simulink model "sim_translation_guidance_law"  (R2024b)
settings: Solver=ode4  StartTime=0.0  StopTime=5000  FixedStep=0.01  RelTol=1e-3
values from neighbouring files (symbols this model uses):
  at_approach = [ax2_t; ay2_t; az2_t]    [guidance_law.m]
  g_moon = 1.62    [guidance_law.m]
  masses = masses(:)    [total_inertia.m]
  r0 = [x0; y0; z0]    [guidance_law.m]
  rt_approach = [x2_t; y2_t; z2_t]    [guidance_law.m]
  rt_breaking = [x1_t; y1_t; z1_t]    [guidance_law.m]
  tgo_approach = 150    [guidance_law.m]
  tgo_breaking = Tgo1    [guidance_law.m]
  v0 = [vx0; vy0; vz0]    [guidance_law.m]
  vt_approach = [vx2_t; vy2_t; vz2_t]    [guidance_law.m]
  vt_breaking = [vx1_t; vy1_t; vz1_t]    [guidance_law.m]
undefined symbols (not defined in the file or in its folder): LLM
libraries: simulink x1
settings Model: NumberOfSteps=2  Creator=gabri  LastModifiedBy=gabri

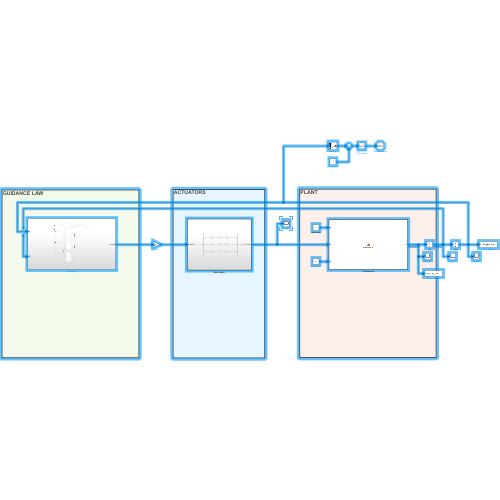
[thumbnail: Simulink's stored preview of the top-level diagram]
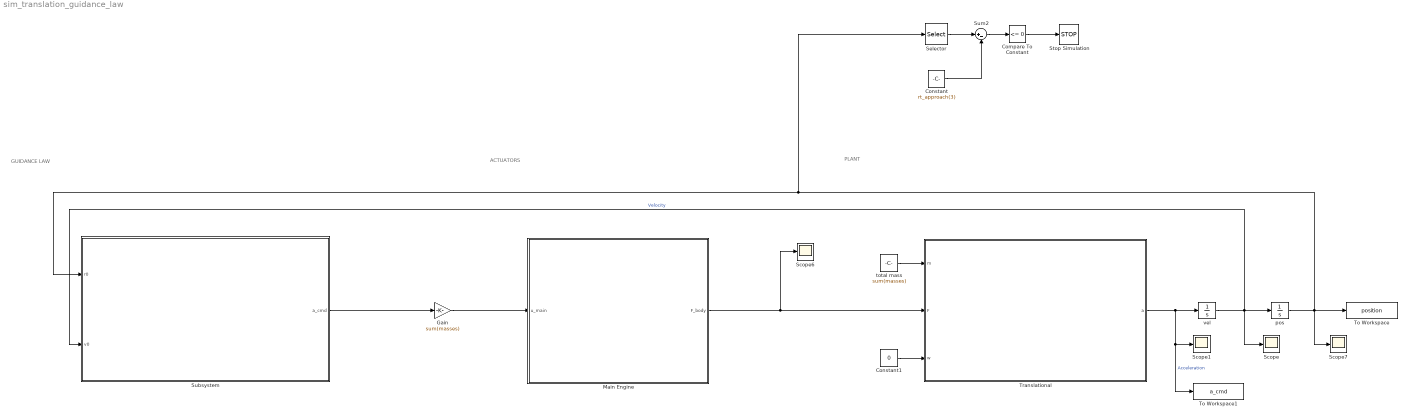
== system sim_translation_guidance_law ==
  note: ACTUATORS
  note: PLANT
  note: GUIDANCE LAW
  Compare To Constant : simulink/Logic and Bit Operations/Compare To Constant  relop=<=  const=0  OutDataTypeStr=boolean
  Constant : Constant  Value=rt_approach(3)
  Constant1 : Constant  Value=0
  Gain : Gain  Gain=sum(masses)
  Main Engine : Subsystem  TreatAsAtomicUnit=on
  Scope{,1,6..7} (4 alike) : Scope
  Selector : Selector  InputPortWidth=3  IndexOptions=Index vector (dialog)  Indices=[3]  OutputSizes=1
  Stop Simulation : Stop
  Subsystem : Subsystem
  Sum2 : Sum  Inputs=|+-
  To Workspace : ToWorkspace  VariableName=position  SampleTime=-1
  To Workspace1 : ToWorkspace  VariableName=a_cmd  SampleTime=-1
  Translational : MATLAB Function  TreatAsAtomicUnit=on
  pos : Integrator  InitialCondition=r0
  total mass : Constant  Value=sum(masses)
  vel : Integrator  InitialCondition=v0
  wires:
  vel/1 -> Subsystem/2(v0), pos/1, Scope/1  "Velocity"
  Main Engine/1(F_body) -> Scope6/1, Translational/2(F)
  Constant1/1 -> Translational/3(w)
  total mass/1 -> Translational/1(m)
  Translational/1(a) -> vel/1, To Workspace1/1, Scope1/1  "Acceleration"
  pos/1 -> Subsystem/1(r0), Selector/1, To Workspace/1, Scope7/1
  Subsystem/1(a_cmd) -> Gain/1
  Gain/1 -> Main Engine/1(u_main)
  Compare To Constant/1 -> Stop Simulation/1
  Sum2/1 -> Compare To Constant/1
  Constant/1 -> Sum2/2
  Selector/1 -> Sum2/1

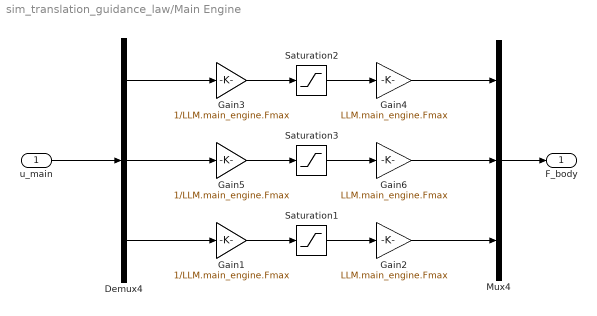
== system sim_translation_guidance_law/Main Engine ==
  u_main : Inport
  Demux4 : Demux  Outputs=3
  Gain1 : Gain  Gain=1/LLM.main_engine.Fmax
  Gain2 : Gain  Gain=LLM.main_engine.Fmax
  Gain3 : Gain  Gain=1/LLM.main_engine.Fmax
  Gain4 : Gain  Gain=LLM.main_engine.Fmax
  Gain5 : Gain  Gain=1/LLM.main_engine.Fmax
  Gain6 : Gain  Gain=LLM.main_engine.Fmax
  Mux4 : Mux  Inputs=3
  Saturation1 : Saturate  UpperLimit=1  LowerLimit=-1
  Saturation2 : Saturate  UpperLimit=1  LowerLimit=-1
  Saturation3 : Saturate  UpperLimit=1  LowerLimit=-1
  F_body : Outport
  wires:
  Demux4/3 -> Gain1/1
  u_main/1 -> Demux4/1
  Mux4/1 -> F_body/1
  Gain2/1 -> Mux4/3
  Saturation1/1 -> Gain2/1
  Gain1/1 -> Saturation1/1
  Gain4/1 -> Mux4/1
  Demux4/1 -> Gain3/1
  Saturation2/1 -> Gain4/1
  Gain3/1 -> Saturation2/1
  Gain6/1 -> Mux4/2
  Demux4/2 -> Gain5/1
  Saturation3/1 -> Gain6/1
  Gain5/1 -> Saturation3/1

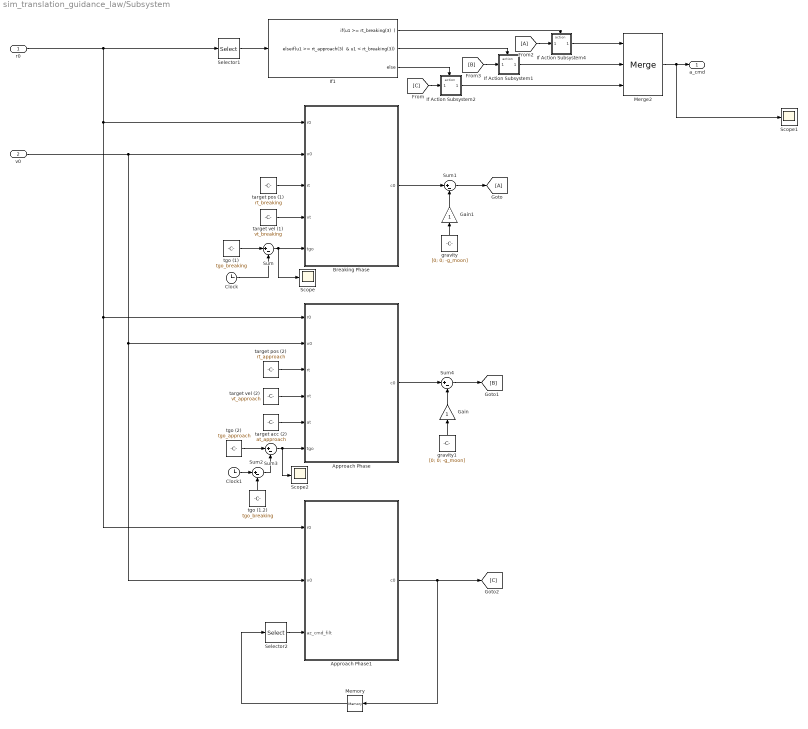
== system sim_translation_guidance_law/Subsystem ==
  r0 : Inport
  v0 : Inport  Port=2
  Approach Phase : MATLAB Function  TreatAsAtomicUnit=on
  Approach Phase1 : MATLAB Function  TreatAsAtomicUnit=on
  Breaking Phase : MATLAB Function  TreatAsAtomicUnit=on
  Clock : Clock
  Clock1 : Clock
  From2 : From
  Gain : Gain
  Gain1 : Gain
  Goto : Goto
  If Action Subsystem1 : Subsystem  TreatAsAtomicUnit=on
  If Action Subsystem2 : Subsystem  TreatAsAtomicUnit=on
  If Action Subsystem4 : Subsystem  TreatAsAtomicUnit=on
  If1 : If  IfExpression=u1 >= rt_breaking(3)  ElseIfExpressions="u1 >= rt_approach(3)  & u1 < rt_breaking(3)"
  Memory : Memory
  Merge2 : Merge  Inputs=3
  Scope : Scope
  Scope1 : Scope
  Scope2 : Scope
  Selector1 : Selector  InputPortWidth=3  IndexOptions=Index vector (dialog)  Indices=[3]  OutputSizes=1
  Selector2 : Selector  InputPortWidth=3  IndexOptions=Index vector (dialog)  Indices=[3]  OutputSizes=1
  Sum{,1..4} (5 alike) : Sum  Inputs=|+-
  gravity : Constant  Value=[0; 0; -g_moon]
  gravity1 : Constant  Value=[0; 0; -g_moon]
  target acc (2) : Constant  Value=at_approach
  target pos (1) : Constant  Value=rt_breaking
  target pos (2) : Constant  Value=rt_approach
  target vel (1) : Constant  Value=vt_breaking
  target vel (2) : Constant  Value=vt_approach
  tgo (1) : Constant  Value=tgo_breaking
  tgo (1.2) : Constant  Value=tgo_breaking
  tgo (2) : Constant  Value=tgo_approach
  a_cmd : Outport
  wires:
  r0/1 -> Approach Phase1/1(r0), Approach Phase/1(r0), Breaking Phase/1(r0), Selector1/1
  v0/1 -> Approach Phase1/2(v0), Approach Phase/2(v0), Breaking Phase/2(v0)
  target vel (1)/1 -> Breaking Phase/4(vt)
  target pos (1)/1 -> Breaking Phase/3(rt)
  Clock/1 -> Sum/2
  tgo (1)/1 -> Sum/1
  Sum/1 -> Scope/1, Breaking Phase/5(tgo)
  Breaking Phase/1(c0) -> Sum1/1
  gravity/1 -> Gain1/1
  Sum1/1 -> Goto/1
  Sum3/1 -> Approach Phase/6(tgo), Scope2/1
  tgo (2)/1 -> Sum3/1
  Selector1/1 -> If1/1
  target pos (2)/1 -> Approach Phase/3(rt)
  target vel (2)/1 -> Approach Phase/4(vt)
  target acc (2)/1 -> Approach Phase/5(at)
  Sum4/1 -> [B]
  Approach Phase/1(c0) -> Sum4/1
  gravity1/1 -> Gain/1
  [B] -> If Action Subsystem1/1(a_cmd)
  From2/1 -> If Action Subsystem4/1(a_cmd)
  If Action Subsystem1/1(Out1) -> Merge2/2
  If Action Subsystem4/1(Out1) -> Merge2/1
  Merge2/1 -> Scope1/1, a_cmd/1
  If1/1 -> If Action Subsystem4/Action
  Clock1/1 -> Sum2/1
  Sum2/1 -> Sum3/2
  tgo (1.2)/1 -> Sum2/2
  If1/2 -> If Action Subsystem1/Action
  If1/3 -> If Action Subsystem2/Action
  If Action Subsystem2/1(a_cmd) -> Merge2/3
  Approach Phase1/1(c0) -> Memory/1, [C]
  [C] -> If Action Subsystem2/1(Input)
  Selector2/1 -> Approach Phase1/3(az_cmd_filt)
  Memory/1 -> Selector2/1
  Gain/1 -> Sum4/2
  Gain1/1 -> Sum1/2

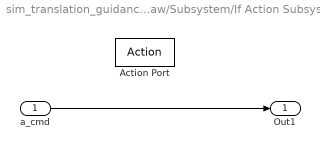
== system sim_translation_guidance_law/Subsystem/If Action Subsystem1 ==
  a_cmd : Inport
  Action Port : ActionPort  ActionPortLabel="elseif(u1 >= rt_approach(3)  & u1 < rt_breaking(3)  )"
  Out1 : Outport
  wires:
  a_cmd/1 -> Out1/1

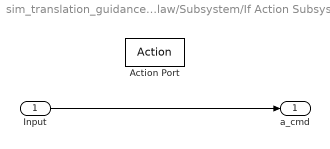
== system sim_translation_guidance_law/Subsystem/If Action Subsystem2 ==
  Input : Inport
  Action Port : ActionPort  ActionPortLabel=else
  a_cmd : Outport
  wires:
  Input/1 -> a_cmd/1

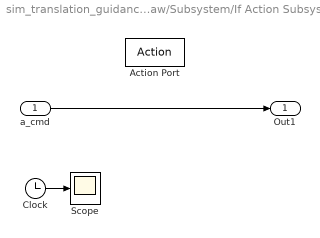
== system sim_translation_guidance_law/Subsystem/If Action Subsystem4 ==
  a_cmd : Inport
  Action Port : ActionPort  ActionPortLabel="if(u1 >= rt_breaking(3)  )"
  Clock : Clock
  Scope : Scope
  Out1 : Outport
  wires:
  a_cmd/1 -> Out1/1
  Clock/1 -> Scope/1

== matlab function sim_translation_guidance_law/Subsystem/Approach Phase ==
  data: r0 input; c0 output; v0 input; rt input; vt input; at input; tgo input
function c0 = approach_coeffs(r0,v0,rt,vt,at,tgo)

    c0 = at - 6*(vt+v0)/tgo + 12*(rt - r0)/(tgo^2);
    if tgo<1
        tgo = 1;
        c0 = [0; 0; -1.63];
    end

end

== matlab function sim_translation_guidance_law/Subsystem/Breaking Phase ==
  data: r0 input; c0 output; v0 input; rt input; vt input; tgo input
function c0 = braking_coeffs(r0, v0, rt, vt, tgo)
    
    c0 = (-2*(vt+2*v0))/tgo + 6*(rt - r0)/(tgo^2);
    if tgo<0.5
        c0 = [0; 0; -1.63];
    end

end

== matlab function sim_translation_guidance_law/Subsystem/Approach Phase1 ==
  data: r0 input; c0 output; v0 input; az_cmd_filt input
function c0 = approach_coeffs(r0,v0,az_cmd_filt)
    
    g_moon  = 1.62;
    az3_cmd = 1.2*g_moon;

    clip = @(u,umin,umax) max(min(u,umax),umin);

    if ~exist('Kxy','var'),      Kxy = 0.8; end
    if ~exist('ax_max','var'),   ax_max = 2.0; end
    if ~exist('ay_max','var'),   ay_max = 2.0; end
    if ~exist('daz_max','var'),  daz_max = 0.6*g_moon; end
    if ~exist('az_cmd_filt','var'), az_cmd_filt = az3_cmd; end
    
    v_td   = -0.1;                 % m/s target at impact
    az_nom = az3_cmd;              % m/s^2 (1.2 g_moon)
    az_max = az_nom + daz_max;     % thrust bound
    a_up_max = max(az_max - g_moon, 0.1);  % net braking capability
    alpha_f  = 0.6;                % smoothing 0..1
    
    % (2) DIVERT table (from your table)
    divert_D   = [25   50    75   100   125   150];      % m
    divert_dT  = [-0.9 -0.6  4.0   8.3   11.1  15.4];    % s
    divert_dDV = [-0.9  0.6  8.2  15.5   20.3  27.4];    % m/s (info)
    
    % Additional remaining time (decreases over time)
    dT_hold = 0;    % s
    dDV_est = 0;    % m/s (optional, for log)
    
    % ================== 1) Horizontal correctors ==================
    if r0(3) > 50
        vx_lim = 10; vy_lim = 10;      % limits under 50 m
        ax_cmd = (abs(v0(1))>vx_lim) * (-Kxy*(abs(v0(1))-vx_lim)*sign(v0(1)));
        ay_cmd = (abs(v0(2))>vy_lim) * (-Kxy*(abs(v0(2))-vy_lim)*sign(v0(2)));
    else
        band = 0.1;                    % deadband ±0.1 m/s under 10 m
        ax_cmd = (v0(1)> band)*(-Kxy*(v0(1)-band)) + (v0(1)<-band)*(-Kxy*(v0(1)+band));
        ay_cmd = (v0(2)> band)*(-Kxy*(v0(2)-band)) + (v0(2)<-band)*(-Kxy*(v0(2)+band));
    end
    ax_cmd = clip(ax_cmd,-ax_max,ax_max);
    ay_cmd = clip(ay_cmd,-ay_max,ay_max);

    % ================== 2) DIVERT management (lateral distance) ========
    D = hypot(r0(1),r0(2));                                   % m
    dT_target = interp1(divert_D, divert_dT, D, 'linear','extrap');
    dDV_target = interp1(divert_D, divert_dDV, D, 'linear','extrap');

    % Never shorten the descent: keep only ΔT>0
    dT_target = max(0, dT_target);
    % Keep the maximum time need observed and consume it progressively
    dT_hold = max(dT_hold, dT_target);
    dDV_est = max(dDV_est, max(0,dDV_target));       % info (not used in loop)

    % Rough estimate of remaining time (used to normalize stretching)
    tgo_est = r0(3) / max(0.5, -v0(3) + 0.1);               % s, robust if vz≈0
    slow_factor = 1 + min(0.8, dT_hold / max(5, tgo_est));   % ≤ +80% on τ

    % ================== 3) Vertical profile v_ref(z) ==================
    v_env = -sqrt(max(v_td^2 + 2*a_up_max*max(r0(3),0), 0));   % stoppable envelope
    if     r0(3) > 200, v_cap = v_env;
    elseif r0(3) > 50,  v_cap = max(v_env, -2);   % intermediate speed limit
    elseif r0(3) > 5,   v_cap = max(v_env, -1);
    else            v_cap = max(v_env, v_td); % converge to -0.2 m/s
    end
    v_ref = v_cap;

    % Base time constant (tighter near ground), then “stretched” by DIVERT
    if     r0(3) > 200, tau = 12.0;
    elseif r0(3) > 100, tau = 6.0;
    elseif r0(3) > 50,  tau = 4.0;
    elseif r0(3) > 20,  tau = 2.0;
    elseif r0(3) > 5,  tau = 1.5;
    else            tau = 2;
    end
    tau = tau * slow_factor;     % <<< buy time for DIVERT

    % Desired net acceleration & commanded thrust
    a_net_des = (v_ref - v0(3))/tau;                   % m/s^2
    az_cmd_raw = g_moon + a_net_des;                % m->thrust
    az_cmd_raw = clip(az_cmd_raw, 0, az_max);
    az_cmd = alpha_f*az_cmd_filt + (1-alpha_f)*az_cmd_raw;
    
    c0 = [ax_cmd; ay_cmd; az_cmd];
    
end

== matlab function sim_translation_guidance_law/Translational ==
  data: m input; F input; a output; w input
function a = translation(m, F, w)

% lunar gravity in inertial frame (verso -Z)
gL = 1.622;
g = [0; 0; -gL];

a = F./m + g;

end
